simulink subsystem "VoltageDriver_SubSystem"  (R2020b)
settings: Solver=VariableStepAuto  StartTime=0.0  StopTime=10.0  RelTol=1e-3
values from neighbouring files (symbols this model uses):
  Ts = 1e-2    (= 0.01)    [balrob_params.m]
undefined symbols (not defined in the file or in its folder): drv
settings Model: Creator=umberto  LastModifiedBy=umberto

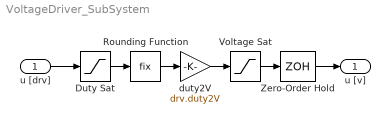
== system VoltageDriver_SubSystem ==
  u [drv] : Inport
  Duty Sat : Saturate  UpperLimit=drv.dutymax  LowerLimit=-drv.dutymax
  Rounding Function : Rounding  Operator=fix
  Voltage Sat : Saturate  UpperLimit=drv.Vbus  LowerLimit=-drv.Vbus
  Zero-Order Hold : ZeroOrderHold  SampleTime=Ts
  duty2V : Gain  Gain=drv.duty2V
  u [v] : Outport
  wires:
  u [drv]/1 -> Duty Sat/1
  Duty Sat/1 -> Rounding Function/1
  Rounding Function/1 -> duty2V/1
  duty2V/1 -> Voltage Sat/1
  Voltage Sat/1 -> Zero-Order Hold/1
  Zero-Order Hold/1 -> u [v]/1
